simulink model "UAV_Dynamics_DataSerialization"  (R2023b)
settings: Solver=ode4  StartTime=0.0  StopTime=10.0  RelTol=1e-3
undefined symbols (not defined in the file): m_to_mm, ms_to_cms, Payload, SampleTime, uT_to_gauss
libraries: uavmavlinklib x7
settings Model: Creator=The MathWorks, Inc.  LastModifiedBy=cardo
settings SolverCC: MaxZcPerStep=1
settings ModelReferenceCC: EnableRefExpFcnMdlSchedulingChecks=on
settings RTWCC: DLArmComputeVersion=19.05

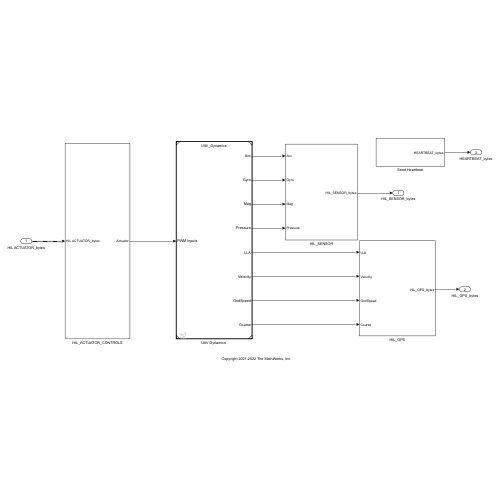
[thumbnail: Simulink's stored preview of the top-level diagram]
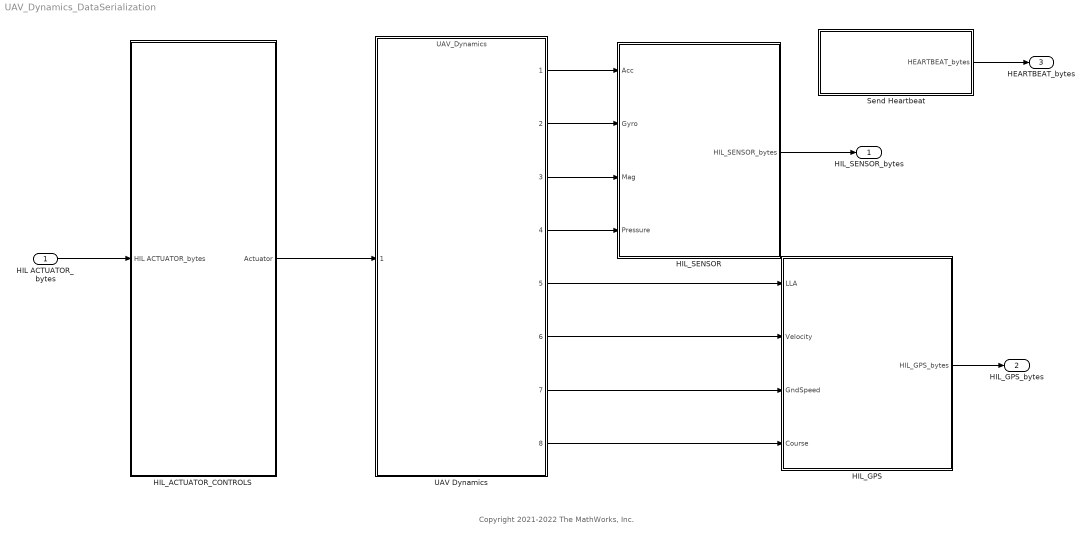
== system UAV_Dynamics_DataSerialization ==
  note: Copyright 2021-2022 The MathWorks, Inc.
  HIL ACTUATOR_bytes : Inport  OutDataTypeStr=uint8  PortDimensions=MAVLink_Input_Read_Size  SampleTime=SampleTime  Interpolate=off
      settings: VarSizeSig=Yes
  HIL_ACTUATOR_CONTROLS : Subsystem
  HIL_GPS : Subsystem
  HIL_SENSOR : Subsystem
  Send Heartbeat : Subsystem
  "UAV Dynamics " : ModelReference  ModelNameDialog=UAV_Dynamics.slx  SimulationMode=Normal  ModelReferenceVersion=4.73
  HIL_SENSOR_bytes : Outport  BusOutputAsStruct=on
  HIL_GPS_bytes : Outport  Port=2  BusOutputAsStruct=on
  HEARTBEAT_bytes : Outport  Port=3  BusOutputAsStruct=on
  wires:
  HIL ACTUATOR_bytes/1 -> HIL_ACTUATOR_CONTROLS/1(HIL ACTUATOR_bytes)
  HIL_ACTUATOR_CONTROLS/1(Actuator) -> "UAV Dynamics "/1
  "UAV Dynamics "/1 -> HIL_SENSOR/1(Acc)
  "UAV Dynamics "/2 -> HIL_SENSOR/2(Gyro)
  "UAV Dynamics "/3 -> HIL_SENSOR/3(Mag)
  "UAV Dynamics "/4 -> HIL_SENSOR/4(Pressure)
  "UAV Dynamics "/8 -> HIL_GPS/4(Course)
  HIL_GPS/1(HIL_GPS_bytes) -> HIL_GPS_bytes/1
  HIL_SENSOR/1(HIL_SENSOR_bytes) -> HIL_SENSOR_bytes/1
  Send Heartbeat/1(HEARTBEAT_bytes) -> HEARTBEAT_bytes/1
  "UAV Dynamics "/5 -> HIL_GPS/1(LLA)
  "UAV Dynamics "/6 -> HIL_GPS/2(Velocity)
  "UAV Dynamics "/7 -> HIL_GPS/3(GndSpeed)

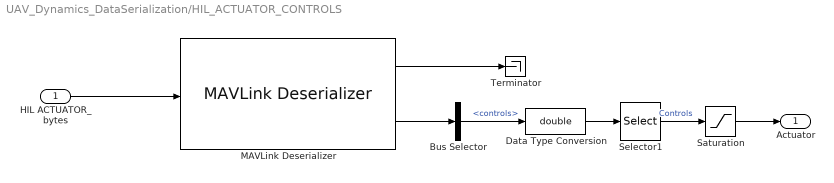
== system UAV_Dynamics_DataSerialization/HIL_ACTUATOR_CONTROLS ==
  HIL ACTUATOR_bytes : Inport
  Bus Selector : BusSelector  OutputSignals=Payload.controls
  Data Type Conversion : DataTypeConversion  OutDataTypeStr=double  SaturateOnIntegerOverflow=off  RndMeth=Floor
  MAVLink Deserializer : uavmavlinklib/MAVLink Deserializer  dialectSource=Select from standard MAVLink dialects  dialect=common.xml  dialectCustom=common.xml  version=2  messageType=HIL_ACTUATOR_CONTROLS  inputDataLength=off  SystemIDFilter=off  systemID=1  ComponentIDFilter=off  componentID=1  queueMsg=off  queueMsgSize=50  dropNum=off
  Saturation : Saturate  UpperLimit=1  LowerLimit=0
  Selector1 : Selector  InputPortWidth=16  IndexOptions=Index vector (dialog)  Indices=[1:4]  OutputSizes=1
  Terminator : Terminator
  Actuator : Outport
  wires:
  Data Type Conversion/1 -> Selector1/1
  MAVLink Deserializer/1 -> Terminator/1
  MAVLink Deserializer/2 -> Bus Selector/1
  Bus Selector/1 -> Data Type Conversion/1  "<controls>"
  HIL ACTUATOR_bytes/1 -> MAVLink Deserializer/1
  Selector1/1 -> Saturation/1  "Controls"
  Saturation/1 -> Actuator/1

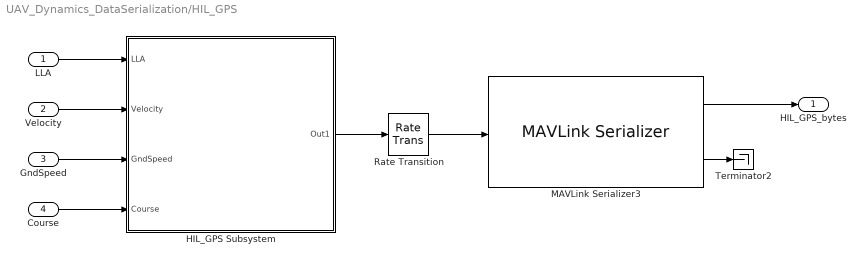
== system UAV_Dynamics_DataSerialization/HIL_GPS ==
  LLA : Inport
  Velocity : Inport  Port=2
  GndSpeed : Inport  Port=3
  Course : Inport  Port=4
  HIL_GPS Subsystem : Subsystem
  MAVLink Serializer3 : uavmavlinklib/MAVLink Serializer  dialectSource=Select from standard MAVLink dialects  dialect=common.xml  dialectCustom=common.xml  version=2  messageType=HIL_GPS
  Rate Transition : RateTransition  OutPortSampleTime=SampleTime
  Terminator2 : Terminator
  HIL_GPS_bytes : Outport
  wires:
  HIL_GPS Subsystem/1(Out1) -> Rate Transition/1
  Course/1 -> HIL_GPS Subsystem/4(Course)
  MAVLink Serializer3/2 -> Terminator2/1
  LLA/1 -> HIL_GPS Subsystem/1(LLA)
  GndSpeed/1 -> HIL_GPS Subsystem/3(GndSpeed)
  MAVLink Serializer3/1 -> HIL_GPS_bytes/1
  Velocity/1 -> HIL_GPS Subsystem/2(Velocity)
  Rate Transition/1 -> MAVLink Serializer3/1

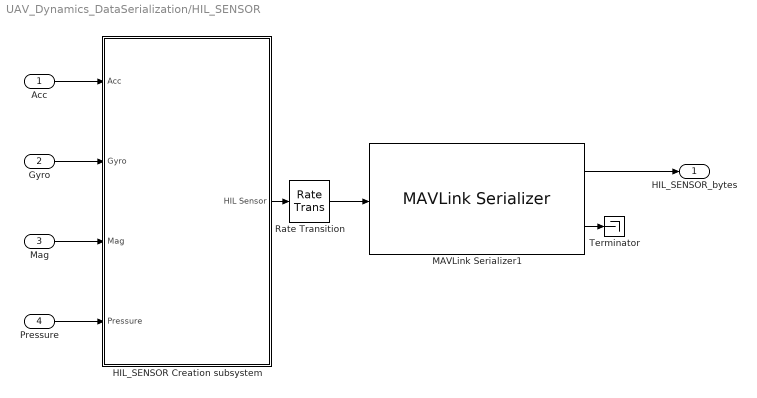
== system UAV_Dynamics_DataSerialization/HIL_SENSOR ==
  Acc : Inport
  Gyro : Inport  Port=2
  Mag : Inport  Port=3
  Pressure : Inport  Port=4
  HIL_SENSOR Creation subsystem : Subsystem
  MAVLink Serializer1 : uavmavlinklib/MAVLink Serializer  dialectSource=Select from standard MAVLink dialects  dialect=common.xml  dialectCustom=common.xml  version=2  messageType=HIL_SENSOR
  Rate Transition : RateTransition  OutPortSampleTime=SampleTime
  Terminator : Terminator
  HIL_SENSOR_bytes : Outport
  wires:
  Pressure/1 -> HIL_SENSOR Creation subsystem/4(Pressure)
  Acc/1 -> HIL_SENSOR Creation subsystem/1(Acc)
  MAVLink Serializer1/2 -> Terminator/1
  MAVLink Serializer1/1 -> HIL_SENSOR_bytes/1
  Mag/1 -> HIL_SENSOR Creation subsystem/3(Mag)
  HIL_SENSOR Creation subsystem/1(HIL Sensor) -> Rate Transition/1
  Gyro/1 -> HIL_SENSOR Creation subsystem/2(Gyro)
  Rate Transition/1 -> MAVLink Serializer1/1

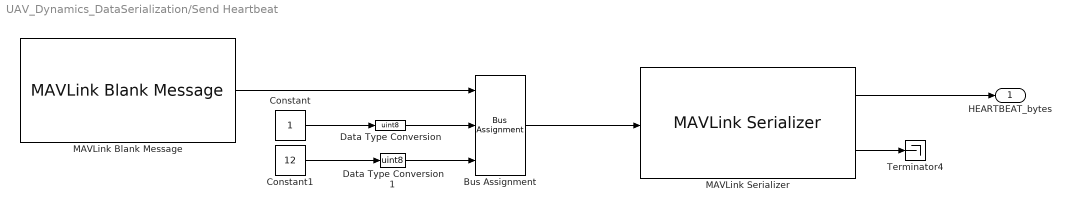
== system UAV_Dynamics_DataSerialization/Send Heartbeat ==
  Bus Assignment : BusAssignment  AssignedSignals=Payload.autopilot,Payload.type
  Constant : Constant  SampleTime=-1
  Constant1 : Constant  Value=12  SampleTime=-1
  Data Type Conversion : DataTypeConversion  OutDataTypeStr=uint8  SaturateOnIntegerOverflow=off  RndMeth=Floor
  Data Type Conversion1 : DataTypeConversion  OutDataTypeStr=uint8  SaturateOnIntegerOverflow=off  RndMeth=Floor
  MAVLink Blank Message : uavmavlinklib/MAVLink Blank Message  dialectSource=Select from standard MAVLink dialects  dialect=common.xml  dialectCustom=common.xml  version=2  messageType=HEARTBEAT  SystemID=2  ComponentID=51  SampleTime=SampleTime
  MAVLink Serializer : uavmavlinklib/MAVLink Serializer  dialectSource=Select from standard MAVLink dialects  dialect=common.xml  dialectCustom=common.xml  version=2  messageType=HEARTBEAT
  Terminator4 : Terminator
  HEARTBEAT_bytes : Outport
  wires:
  Bus Assignment/1 -> MAVLink Serializer/1
  Constant/1 -> Data Type Conversion/1
  MAVLink Serializer/1 -> HEARTBEAT_bytes/1
  Data Type Conversion1/1 -> Bus Assignment/3
  Data Type Conversion/1 -> Bus Assignment/2
  MAVLink Serializer/2 -> Terminator4/1
  Constant1/1 -> Data Type Conversion1/1
  MAVLink Blank Message/1 -> Bus Assignment/1

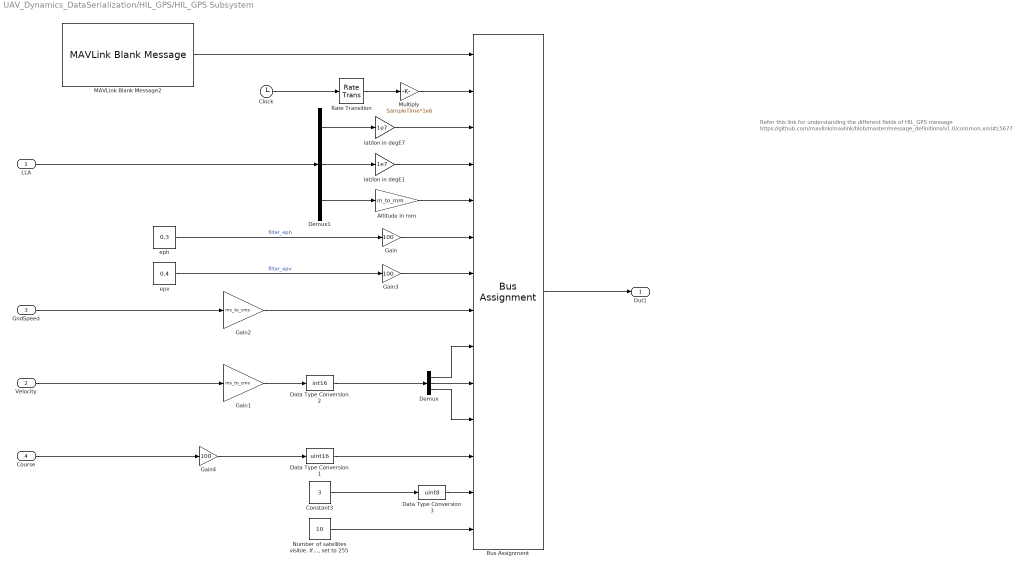
== system UAV_Dynamics_DataSerialization/HIL_GPS/HIL_GPS Subsystem ==
  note: Refer this link for understanding the different fields of HIL_GPS message https://github.com/mavlink/mavlink/blob/master/message_definitions/v1.0/common.xml#L5677
  LLA : Inport
  Velocity : Inport  Port=2
  GndSpeed : Inport  Port=3
  Course : Inport  Port=4
  Altitude in mm : Gain  Gain=m_to_mm  OutDataTypeStr=Inherit: Inherit via back propagation
  Bus Assignment : BusAssignment  AssignedSignals=Payload.time_usec,Payload.lat,Payload.lon,Payload.alt,Payload.eph,Payload.epv,Payload.vel,Payload.vn,Payload.ve,Payload.vd,Payload.cog,Payload.fix_type,Payload.satellites_visible
  Clock : Clock
  Constant3 : Constant  Value=3  OutDataTypeStr=Inherit: Inherit via back propagation  SampleTime=-1
  Data Type Conversion1 : DataTypeConversion  OutDataTypeStr=uint16  SaturateOnIntegerOverflow=off  RndMeth=Floor
  Data Type Conversion2 : DataTypeConversion  OutDataTypeStr=int16  SaturateOnIntegerOverflow=off  RndMeth=Floor
  Data Type Conversion3 : DataTypeConversion  OutDataTypeStr=uint8  SaturateOnIntegerOverflow=off  RndMeth=Floor
  Demux : Demux  Outputs=3
  Demux1 : Demux  Outputs=3
  Gain : Gain  Gain=100  OutDataTypeStr=Inherit: Inherit via back propagation
  Gain1 : Gain  Gain=ms_to_cms
  Gain2 : Gain  Gain=ms_to_cms  OutDataTypeStr=uint16
  Gain3 : Gain  Gain=100  OutDataTypeStr=Inherit: Inherit via back propagation
  Gain4 : Gain  Gain=100
  MAVLink Blank Message2 : uavmavlinklib/MAVLink Blank Message  dialectSource=Select from standard MAVLink dialects  dialect=common.xml  dialectCustom=common.xml  version=2  messageType=HIL_GPS  SystemID=2  ComponentID=51  SampleTime=SampleTime
  Multiply : Gain  Gain=SampleTime*1e6  OutDataTypeStr=Inherit: Inherit via back propagation
  "Number of satellites visible. If unknown, set to 255" : Constant  Value=10  OutDataTypeStr=Inherit: Inherit via back propagation  SampleTime=-1
  Rate Transition : RateTransition
  eph : Constant  Value=0.3  SampleTime=-1
  epv : Constant  Value=0.4  SampleTime=-1
  lat/lon in degE1 : Gain  Gain=1e7  OutDataTypeStr=Inherit: Inherit via back propagation
  lat/lon in degE7 : Gain  Gain=1e7  OutDataTypeStr=Inherit: Inherit via back propagation
  Out1 : Outport
  wires:
  Gain2/1 -> Bus Assignment/8
  lat/lon in degE7/1 -> Bus Assignment/3
  Demux1/1 -> lat/lon in degE7/1
  Demux/3 -> Bus Assignment/11
  MAVLink Blank Message2/1 -> Bus Assignment/1
  Gain1/1 -> Data Type Conversion2/1
  Demux1/3 -> Altitude in mm/1
  Demux1/2 -> lat/lon in degE1/1
  Demux/1 -> Bus Assignment/9
  lat/lon in degE1/1 -> Bus Assignment/4
  Altitude in mm/1 -> Bus Assignment/5
  Data Type Conversion2/1 -> Demux/1
  Demux/2 -> Bus Assignment/10
  Bus Assignment/1 -> Out1/1
  "Number of satellites visible. If unknown, set to 255"/1 -> Bus Assignment/14
  Gain/1 -> Bus Assignment/6
  Gain3/1 -> Bus Assignment/7
  LLA/1 -> Demux1/1
  GndSpeed/1 -> Gain2/1
  Velocity/1 -> Gain1/1
  Course/1 -> Gain4/1
  Data Type Conversion1/1 -> Bus Assignment/12
  eph/1 -> Gain/1  "filter_eph"
  epv/1 -> Gain3/1  "filter_epv"
  Data Type Conversion3/1 -> Bus Assignment/13
  Gain4/1 -> Data Type Conversion1/1
  Constant3/1 -> Data Type Conversion3/1
  Clock/1 -> Rate Transition/1
  Rate Transition/1 -> Multiply/1
  Multiply/1 -> Bus Assignment/2

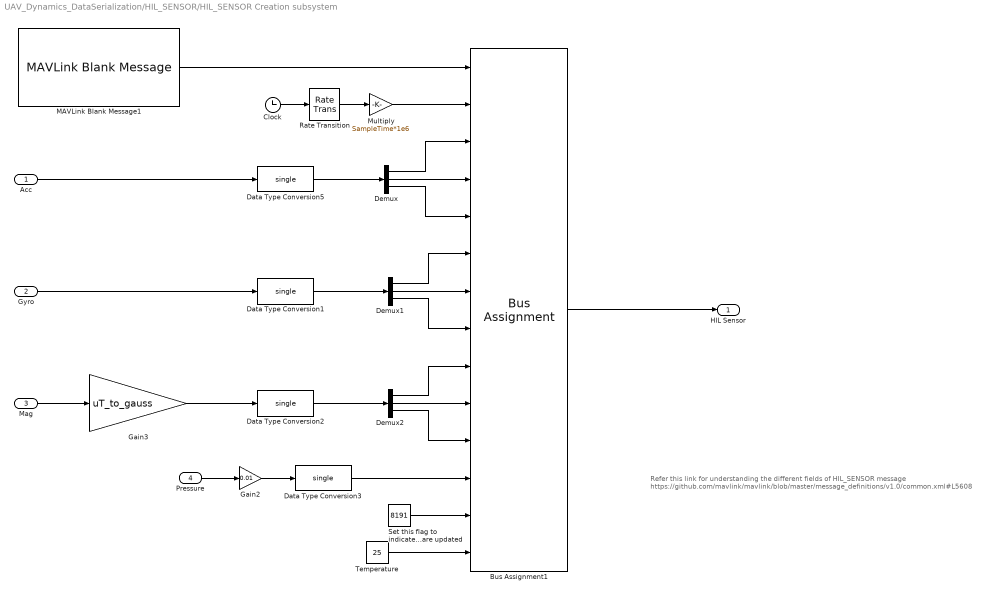
== system UAV_Dynamics_DataSerialization/HIL_SENSOR/HIL_SENSOR Creation subsystem ==
  note: Refer this link for understanding the different fields of HIL_SENSOR message https://github.com/mavlink/mavlink/blob/master/message_definitions/v1.0/common.xml#L5608
  Acc : Inport
  Gyro : Inport  Port=2
  Mag : Inport  Port=3
  Pressure : Inport  Port=4
  Bus Assignment1 : BusAssignment  AssignedSignals=Payload.time_usec,Payload.xacc,Payload.yacc,Payload.zacc,Payload.xgyro,Payload.ygyro,Payload.zgyro,Payload.xmag,Payload.ymag,Payload.zmag,Payload.abs_pressure,Payload.fields_updated,Payload.temperature
  Clock : Clock
  Data Type Conversion{1..3,5} (4 alike) : DataTypeConversion  OutDataTypeStr=single  SaturateOnIntegerOverflow=off  RndMeth=Floor
  Demux : Demux  Outputs=3
  Demux1 : Demux  Outputs=3
  Demux2 : Demux  Outputs=3
  Gain2 : Gain  Gain=0.01  OutDataTypeStr=single
  Gain3 : Gain  Gain=uT_to_gauss
  MAVLink Blank Message1 : uavmavlinklib/MAVLink Blank Message  dialectSource=Select from standard MAVLink dialects  dialect=common.xml  dialectCustom=common.xml  version=2  messageType=HIL_SENSOR  SystemID=2  ComponentID=51  SampleTime=SampleTime
  Multiply : Gain  Gain=SampleTime*1e6  OutDataTypeStr=Inherit: Inherit via back propagation
  Rate Transition : RateTransition
  Set this flag to indicate all flags are updated : Constant  Value=8191  OutDataTypeStr=Inherit: Inherit via back propagation  SampleTime=-1
  Temperature : Constant  Value=25  OutDataTypeStr=Inherit: Inherit via back propagation  SampleTime=-1
  HIL Sensor : Outport
  wires:
  Data Type Conversion2/1 -> Demux2/1
  Demux1/1 -> Bus Assignment1/6
  Mag/1 -> Gain3/1
  Demux1/3 -> Bus Assignment1/8
  Data Type Conversion1/1 -> Demux1/1
  Gyro/1 -> Data Type Conversion1/1
  Bus Assignment1/1 -> HIL Sensor/1
  Demux/3 -> Bus Assignment1/5
  Demux2/2 -> Bus Assignment1/10
  Demux2/3 -> Bus Assignment1/11
  Data Type Conversion5/1 -> Demux/1
  Demux/1 -> Bus Assignment1/3
  MAVLink Blank Message1/1 -> Bus Assignment1/1
  Demux2/1 -> Bus Assignment1/9
  Demux/2 -> Bus Assignment1/4
  Demux1/2 -> Bus Assignment1/7
  Acc/1 -> Data Type Conversion5/1
  Data Type Conversion3/1 -> Bus Assignment1/12
  Gain3/1 -> Data Type Conversion2/1
  Set this flag to indicate all flags are updated/1 -> Bus Assignment1/13
  Pressure/1 -> Gain2/1
  Clock/1 -> Rate Transition/1
  Rate Transition/1 -> Multiply/1
  Multiply/1 -> Bus Assignment1/2
  Gain2/1 -> Data Type Conversion3/1
  Temperature/1 -> Bus Assignment1/14
